simulink model "Buck_Boost"  (R2020a)
settings: Solver=VariableStepAuto  StartTime=0.0  StopTime=10.0  RelTol=1e-3
undefined symbols (not defined in the file): C, d, L, R
settings Model: Creator=Husnain Awan  LastModifiedBy=Husnain Awan

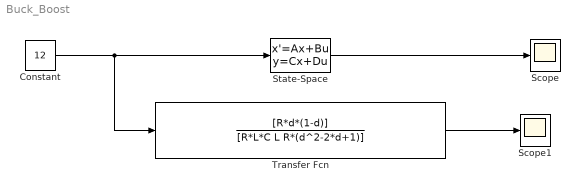
== system Buck_Boost ==
  Constant : Constant  Value=12
  Scope : Scope
  Scope1 : Scope
  State-Space : StateSpace  A=[-1/(R*C) (1-d)/C; (d-1)/L 0]  B=[0;d/L]  C=[1 0]  D=0  InitialCondition=0
  Transfer Fcn : TransferFcn  Numerator=[R*d*(1-d)]  Denominator=[R*L*C L R*(d^2-2*d+1)]
  wires:
  Constant/1 -> Transfer Fcn/1, State-Space/1
  State-Space/1 -> Scope/1
  Transfer Fcn/1 -> Scope1/1
